simulink model "pend_m"  (R2022a)
settings: Solver=FixedStepAuto  StartTime=0.0  StopTime=SIM_TIME  FixedStep=STEP_SIZE  RelTol=1e-3
undefined symbols (not defined in the file): a_st, bm, c, FN, g, I, Jm, ke, kt, l, Lm, M, m, mu_k, mu_s, mu_v, r, Rm, theta0, theta_dot0, x0, x_dot0
settings Model: Creator=farfar  LastModifiedBy=farfar
settings DataIOCC: ReturnWorkspaceOutputs=off

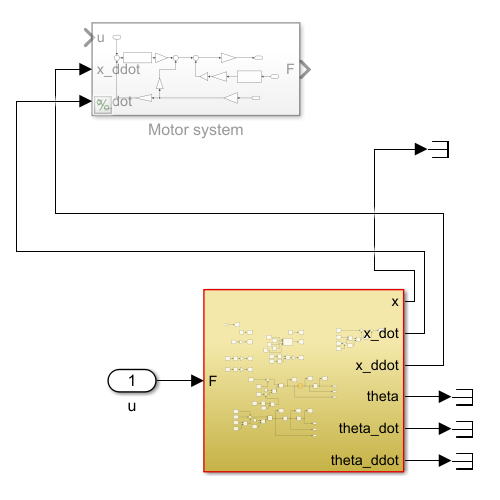
[thumbnail: Simulink's stored preview of the top-level diagram]
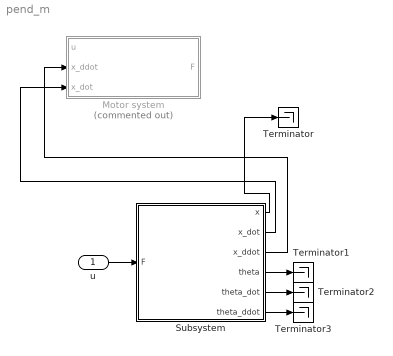
== system pend_m ==
  u : Inport
  Motor system : Subsystem  Commented=on
  Subsystem : Subsystem
  Terminator{,1..3} (4 alike) : Terminator
  wires:
  Subsystem/2(x_dot) -> Motor system/3(x_dot)
  Subsystem/3(x_ddot) -> Motor system/2(x_ddot)
  Subsystem/6(theta_ddot) -> Terminator3/1
  Subsystem/5(theta_dot) -> Terminator2/1
  Subsystem/4(theta) -> Terminator1/1
  Subsystem/1(x) -> Terminator/1
  u/1 -> Subsystem/1(F)

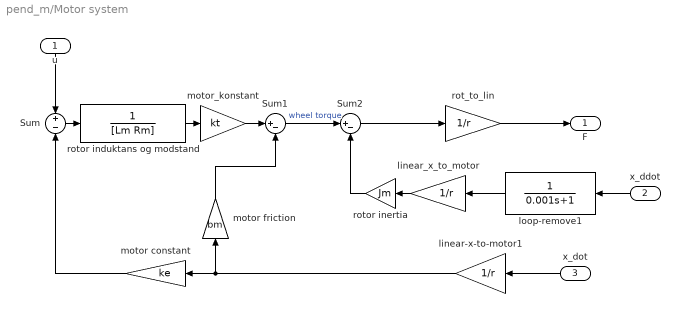
== system pend_m/Motor system ==
  u : Inport
  x_ddot : Inport  Port=2
  x_dot : Inport  Port=3
  Sum : Sum  Inputs=+|-
  Sum1 : Sum  Inputs=|+-
  Sum2 : Sum  Inputs=|+-
  linear-x-to-motor1 : Gain  Gain=1/r
  linear_x_to_motor : Gain  Gain=1/r
  loop-remove1 : TransferFcn  Denominator=[0.001 1]
  motor constant : Gain  Gain=ke
  motor friction : Gain  Gain=bm
  motor_konstant : Gain  Gain=kt
  rot_to_lin : Gain  Gain=1/r
  rotor induktans og modstand : TransferFcn  Denominator=[Lm Rm]
  rotor inertia : Gain  Gain=Jm
  F : Outport
  wires:
  linear-x-to-motor1/1 -> motor constant/1, motor friction/1
  rotor induktans og modstand/1 -> motor_konstant/1
  u/1 -> Sum/1
  linear_x_to_motor/1 -> rotor inertia/1
  Sum2/1 -> rot_to_lin/1
  x_dot/1 -> linear-x-to-motor1/1
  rot_to_lin/1 -> F/1
  x_ddot/1 -> loop-remove1/1
  Sum/1 -> rotor induktans og modstand/1
  motor constant/1 -> Sum/2
  Sum1/1 -> Sum2/1  "wheel torque"
  rotor inertia/1 -> Sum2/2
  motor friction/1 -> Sum1/2
  motor_konstant/1 -> Sum1/1
  loop-remove1/1 -> linear_x_to_motor/1

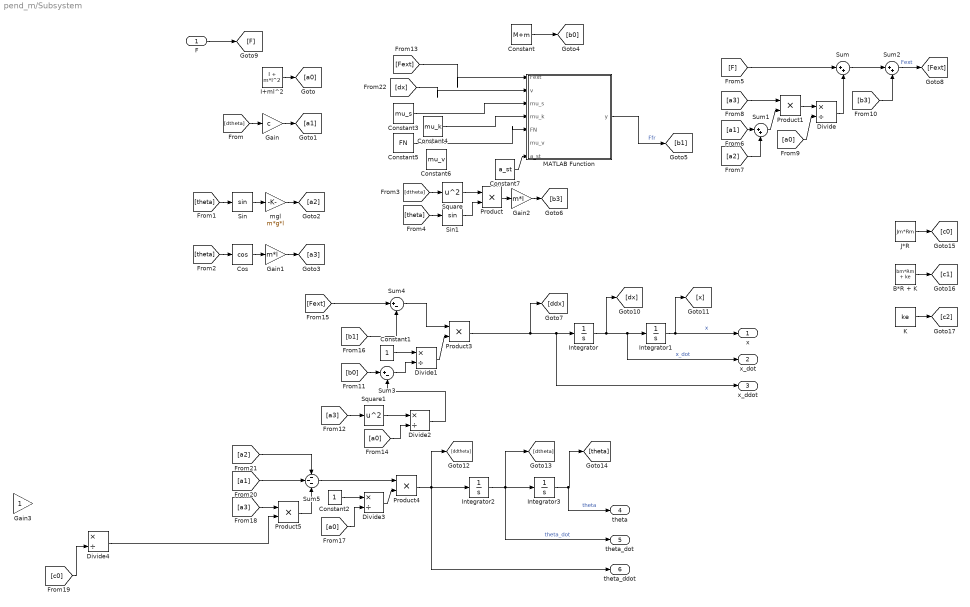
== system pend_m/Subsystem ==
  F : Inport
  B*R + K : Constant  Value=bm*Rm + ke
  Constant : Constant  Value=M+m
  Constant1 : Constant
  Constant2 : Constant
  Constant3 : Constant  Value=mu_s
  Constant4 : Constant  Value=mu_k
  Constant5 : Constant  Value=FN
  Constant6 : Constant  Value=mu_v
  Constant7 : Constant  Value=a_st
  Cos : Trigonometry  Operator=cos
  Divide{,1..4} (5 alike) : Product  Inputs=*/
  Gain : Gain  Gain=c
  Gain1 : Gain  Gain=m*l
  Gain2 : Gain  Gain=m*l
  Gain3 : Gain
  I+ml^2 : Constant  Value=I + m*l^2
  Integrator : Integrator  InitialCondition=x_dot0
  Integrator1 : Integrator  InitialCondition=x0
  Integrator2 : Integrator  InitialCondition=theta_dot0
  Integrator3 : Integrator  InitialCondition=theta0
  J*R : Constant  Value=Jm*Rm
  K : Constant  Value=ke
  MATLAB Function : MATLAB Function  TreatAsAtomicUnit=on
  Product{,1,3..5} (5 alike) : Product
  Sin : Trigonometry
  Sin1 : Trigonometry
  Square : Math  Operator=square
  Square1 : Math  Operator=square
  Sum : Sum  Inputs=|++
  Sum1 : Sum  Inputs=|++
  Sum2 : Sum  Inputs=|++
  Sum3 : Sum  Inputs=|+-
  Sum4 : Sum  Inputs=|+-
  Sum5 : Sum  Inputs=---
  mgl : Gain  Gain=m*g*l
  x : Outport
  x_dot : Outport  Port=2
  x_ddot : Outport  Port=3
  theta : Outport  Port=4
  theta_dot : Outport  Port=5
  theta_ddot : Outport  Port=6
  wires:
  Product4/1 -> theta_ddot/1, Integrator2/1, [ddtheta]
  Integrator/1 -> [dx], x_dot/1, Integrator1/1  "x_dot"
  Constant/1 -> [b0]
  I+ml^2/1 -> [a0]
  [theta] -> Sin/1
  [a1] -> Sum5/2
  Product1/1 -> Divide/1
  [dtheta] -> Gain/1
  mgl/1 -> [a2]
  [F] -> Sum/1
  [a3] -> Square1/1
  Sin1/1 -> Product/2
  [theta] -> Cos/1
  Gain/1 -> [a1]
  [dx] -> MATLAB Function/2(v)
  F/1 -> [F]
  [a0] -> Divide3/2
  [a0] -> Divide2/2
  Cos/1 -> Gain1/1
  Sum3/1 -> Divide1/2
  Divide3/1 -> Product4/2
  Square/1 -> Product/1
  [a0] -> Divide/2
  Sum5/1 -> Product4/1
  [b3] -> Sum2/2
  MATLAB Function/1(y) -> [b1]  "Ffr"
  [a1] -> Sum1/1
  Product/1 -> Gain2/1
  Gain1/1 -> [a3]
  Sum2/1 -> [Fext]  "Fext"
  [dtheta] -> Square/1
  Constant4/1 -> MATLAB Function/4(mu_k)
  [a2] -> Sum1/2
  Constant1/1 -> Divide1/1
  Divide/1 -> Sum/2
  Constant2/1 -> Divide3/1
  Sum4/1 -> Product3/1
  Divide2/1 -> Sum3/2
  Sin/1 -> mgl/1
  Divide1/1 -> Product3/2
  Gain2/1 -> [b3]
  [a3] -> Product5/1
  Integrator3/1 -> theta/1, [theta]  "theta"
  Integrator2/1 -> theta_dot/1, [dtheta], Integrator3/1  "theta_dot"
  [b1] -> Sum4/2
  [a3] -> Product1/1
  Square1/1 -> Divide2/1
  Constant3/1 -> MATLAB Function/3(mu_s)
  [b0] -> Sum3/1
  Constant5/1 -> MATLAB Function/5(FN)
  Sum/1 -> Sum2/1
  Product5/1 -> Sum5/3
  Integrator1/1 -> x/1, [x]  "x"
  [Fext] -> Sum4/1
  [a2] -> Sum5/1
  Divide4/1 -> Product5/2
  [theta] -> Sin1/1
  Sum1/1 -> Product1/2
  [Fext] -> MATLAB Function/1(Fext)
  Constant7/1 -> MATLAB Function/7(a_st)
  Product3/1 -> x_ddot/1, Integrator/1, [ddx]
  J*R/1 -> [c0]
  B*R + K/1 -> [c1]
  K/1 -> [c2]
  [c0] -> Divide4/2

== matlab function pend_m/Subsystem/MATLAB Function ==
  data: Fext input; y output; v input; mu_s input; mu_k input; FN input; mu_v input; a_st input
function y = fcn(Fext, v, mu_s, mu_k, FN, mu_v, a_st)
%mu_s = 1.5;
%mu_k = 0.5;
%mu_v = 0.3;
%a_st = 1;
%FN = 10*9.8;
Fs = mu_s * FN;% * sign(v);
Fk = mu_k * FN;% * sign(v);
Fv = 0;%mu_v * FN;

v_tol = 0.00000000000000001;
y = 0;
opt = 0;
if and(abs(v) <= v_tol, Fext < Fs)
    y = Fext;
    opt = 1;
elseif and(abs(v) <= v_tol, Fext >= Fs)
    y = Fs;
    opt = 2;
elseif and(abs(v) > v_tol, v > 0)
    y = Fk + (Fs - Fk)*exp(-a_st * v) + Fv * v;
    opt = 3;
elseif and(abs(v) > v_tol, v < 0) 
    y = -Fk + (Fk - Fs)*exp(a_st * v) - Fv * v;
    opt = 4;
end
